simulink model "CompFeatures"  (R2012b)
settings: Solver=FixedStepDiscrete  StartTime=0.0  StopTime=50  RelTol=1e-3
undefined symbols (not defined in the file): gcbh, rmidispblock
settings Model: RequirementInfo={'other' '..\..\..\requirements\ebd_srs.doc' '@Simulink_requirement_item_4' 'true' 'REQ001- Filter input signal via polyphase digital filter bank' 'Requirement' } %GIDa_bfa4a348_cd9f_4101_a776_3ea215f34dae  RecordCoverage=on  Creator=aanantha  LastModifiedBy=klindqvi
settings DataIOCC: SaveFormat=Structure  SignalLoggingSaveFormat=ModelDataLogs  SaveOutput=off  SaveTime=off  SignalLoggingName=logsOut
settings OptimizationCC: InlineParams=on  OptimizeModelRefInitCode=on  LifeSpan=1
settings DebuggingCC: ReadBeforeWriteMsg=DisableAll  WriteAfterWriteMsg=DisableAll  WriteAfterReadMsg=DisableAll  SolverPrmCheckMsg=none  InheritedTsInSrcMsg=none  ParameterPrecisionLossMsg=none  FcnCallInpInsideContextMsg=EnableAllAsWarning
settings HardwareCC: ProdLargestAtomicInteger=Long  ProdLargestAtomicFloat=Double  ProdEndianess=LittleEndian  ProdHWDeviceType=ARM Compatible->ARM Cortex
settings RTWCC: SystemTargetFile=ert.tlc  TemplateMakefile=ert_default_tmf  Description=Embedded Coder  GenerateReport=on  RTWVerbose=off  ProcessScript=ert_make_rtw_hook  IncludeHyperlinkInReport=on  LaunchReport=on  PortableWordSizes=on  CodeProfilingSaveOptions=AllData  GenerateTraceInfo=on  GenerateTraceReportSl=on  GenerateTraceReportSf=on  GenerateTraceReportEml=on  GenerateCodeMetricsReport=on
settings CodeAppCC: IgnoreCustomStorageClasses=off
settings ERTTargetCC: CodeReplacementLibrary=GCC ARM Cortex-A8  MultiwordLength=2048  GenerateSampleERTMain=on  ERTCustomFileTemplate=example_file_process.tlc  ConvertIfToSwitch=off  SuppressUnreachableDefaultCases=off

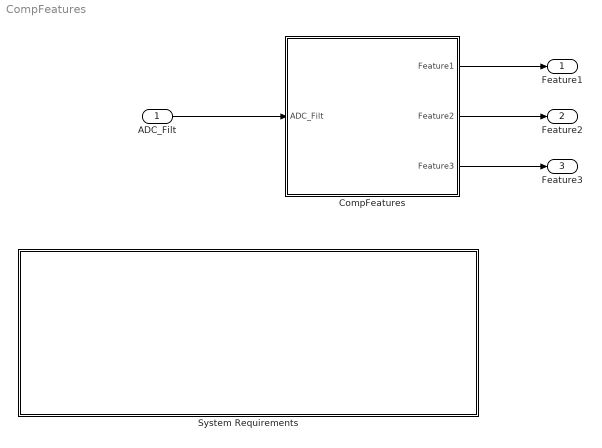
== system CompFeatures ==
  ADC_Filt : Inport  OutDataTypeStr=single  PortDimensions=4  SampleTime=[0.089,0]
  CompFeatures : Subsystem
  System Requirements : Subsystem  LoadFcn=rmidispblock('load',gcbh)  mask(System Requirements){id=SystemReq, title=System Requirements}
      mask prompts: title "Block Title"
      mask help: Lists the requirements for the current model.
      mask init:
      | id = 'SystemReq';
      | [w,h] = rmidispblock('display',gcbh);
      settings: CopyFcn=rmidispblock('create',gcbh)  DeleteFcn=rmidispblock('delete',gcbh)  ModelCloseFcn=rmidispblock('close',gcbh)  PreSaveFcn=rmidispblock('close',gcbh)  PostSaveFcn=rmidispblock('open',gcbh)  OpenFcn=rmidispblock('open',gcbh)  MoveFcn=rmidispblock('move',gcbh)
      mask Help: helpview(fullfile(docroot,'toolbox','slvnv','slvnv.map'),'systemrequirements')
      mask Display: text(w/2,h-4,rmidispblock('title',gcbh),'horizontalAlignment','center','verticalAlignment','top')
  Feature1 : Outport  OutDataTypeStr=single  PortDimensions=1  SampleTime=[0.08900000000000001,0]
  Feature2 : Outport  Port=2  OutDataTypeStr=single  PortDimensions=1  SampleTime=[0.08900000000000001,0]
  Feature3 : Outport  Port=3  OutDataTypeStr=single  PortDimensions=1  SampleTime=[0.08900000000000001,0]
  wires:
  ADC_Filt/1 -> CompFeatures/1(ADC_Filt)
  CompFeatures/1(Feature1) -> Feature1/1
  CompFeatures/2(Feature2) -> Feature2/1
  CompFeatures/3(Feature3) -> Feature3/1

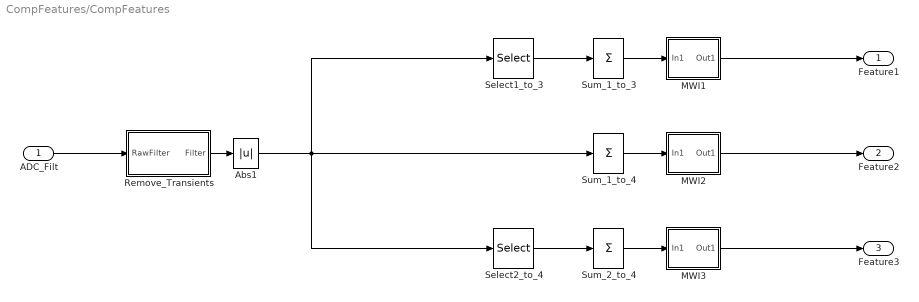
== system CompFeatures/CompFeatures ==
  ADC_Filt : Inport
  Abs1 : Abs
  MWI1 : Subsystem  RequirementInfo={'other' '..\..\..\requirements\ebd_srs.doc' '@Simulink_requirement_MWI' 'true' 'The computed sums of filter bank outputs are all passed through Moving Window Integrators that averages the current and previous value.' '' } %GIDa_3cd60982_fe68_4a22_829b_cdbc47747a6e
  MWI2 : Subsystem  RequirementInfo={'other' '..\..\..\requirements\ebd_srs.doc' '@Simulink_requirement_MWI' 'true' 'The computed sums of filter bank outputs are all passed through Moving Window Integrators that averages the current and previous value.' '' } %GIDa_66a30cf9_fe2b_486a_8212_cb7a33acd1ee
  MWI3 : Subsystem  RequirementInfo={'other' '..\..\..\requirements\ebd_srs.doc' '@Simulink_requirement_MWI' 'true' 'The computed sums of filter bank outputs are all passed through Moving Window Integrators that averages the current and previous value.' '' } %GIDa_a2fc5531_f324_49da_86f2_4acd55f4c339
  Remove_Transients : Subsystem
  Select1_to_3 : Selector  InputPortWidth=4  IndexOptions=Index vector (dialog)  Indices=[1 2 3]  OutputSizes=1
  Select2_to_4 : Selector  InputPortWidth=4  IndexOptions=Index vector (dialog)  Indices=[2 3 4]  OutputSizes=1
  Sum_1_to_3 : Sum  Inputs=+
  Sum_1_to_4 : Sum  Inputs=+
  Sum_2_to_4 : Sum  Inputs=+
  Feature1 : Outport
  Feature2 : Outport  Port=2
  Feature3 : Outport  Port=3
  wires:
  ADC_Filt/1 -> Remove_Transients/1(RawFilter)
  Remove_Transients/1(Filter) -> Abs1/1
  MWI2/1(Out1) -> Feature2/1
  MWI3/1(Out1) -> Feature3/1
  Sum_1_to_4/1 -> MWI2/1(In1)
  Sum_2_to_4/1 -> MWI3/1(In1)
  Select1_to_3/1 -> Sum_1_to_3/1
  Sum_1_to_3/1 -> MWI1/1(In1)
  Select2_to_4/1 -> Sum_2_to_4/1
  Abs1/1 -> Sum_1_to_4/1, Select1_to_3/1, Select2_to_4/1
  MWI1/1(Out1) -> Feature1/1

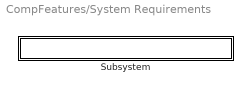
== system CompFeatures/System Requirements ==
  Subsystem : Subsystem  mask{label=0, index=1}
      mask init:
      | label = rmidispblock('label',index);
      settings: OpenFcn=rmidispblock('openReq',gcbh);
      mask Display: text(0,0,label,'horizontalAlignment','left','verticalAlignment','bottom')

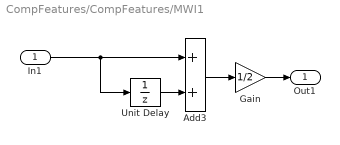
== system CompFeatures/CompFeatures/MWI1 ==
  In1 : Inport
  Add3 : Sum  Inputs=2
  Gain : Gain  Gain=1/2  OutDataTypeStr=Inherit: Inherit via back propagation
  Unit Delay : UnitDelay  SampleTime=-1
  Out1 : Outport
  wires:
  In1/1 -> Unit Delay/1, Add3/1
  Unit Delay/1 -> Add3/2
  Add3/1 -> Gain/1
  Gain/1 -> Out1/1

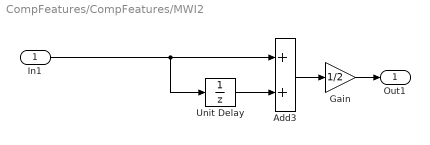
== system CompFeatures/CompFeatures/MWI2 ==
  In1 : Inport
  Add3 : Sum  Inputs=2
  Gain : Gain  Gain=1/2
  Unit Delay : UnitDelay  SampleTime=-1
  Out1 : Outport
  wires:
  Gain/1 -> Out1/1
  Add3/1 -> Gain/1
  Unit Delay/1 -> Add3/2
  In1/1 -> Add3/1, Unit Delay/1

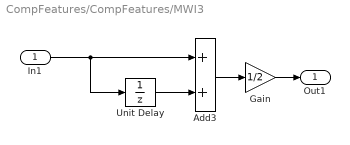
== system CompFeatures/CompFeatures/MWI3 ==
  In1 : Inport
  Add3 : Sum  Inputs=2
  Gain : Gain  Gain=1/2
  Unit Delay : UnitDelay  SampleTime=-1
  Out1 : Outport
  wires:
  In1/1 -> Unit Delay/1, Add3/1
  Unit Delay/1 -> Add3/2
  Add3/1 -> Gain/1
  Gain/1 -> Out1/1

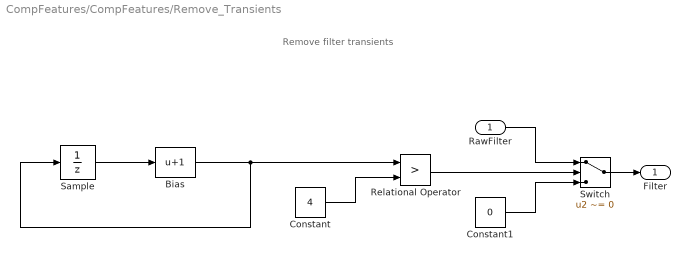
== system CompFeatures/CompFeatures/Remove_Transients ==
  note: Remove filter transients
  RawFilter : Inport
  Bias : Bias  Bias=1
  Constant : Constant  Value=4
  Constant1 : Constant  Value=0  OutDataTypeStr=single
  Relational Operator : RelationalOperator  Operator=>  OutDataTypeStr=boolean
  Sample : UnitDelay  SampleTime=-1
  Switch : Switch  Criteria=u2 ~= 0
  Filter : Outport
  wires:
  Sample/1 -> Bias/1
  Bias/1 -> Sample/1, Relational Operator/1
  Constant/1 -> Relational Operator/2
  Relational Operator/1 -> Switch/2
  RawFilter/1 -> Switch/1
  Constant1/1 -> Switch/3
  Switch/1 -> Filter/1

== system CompFeatures/System Requirements/Subsystem ==
